simulink model "SimPIDdir2020b"  (R2021b)
settings: Solver=VariableStepAuto  StartTime=0.0  StopTime=15  RelTol=1e-3
values from neighbouring files (symbols this model uses):
  g_r = tf(Mod_r)    [dirPID.m]
  Kd = 1.5    [dirPID.m]
  Ki = 0.005    [dirPID.m]
  Kp = 5    [dirPID.m]
libraries: slpidlib x2, simulink x1
settings Model: Creator=danie  LastModifiedBy=Daniel
settings SolverCC: AlgebraicLoopSolver=TrustRegion
settings DebuggingCC: UnconnectedInputMsg=none  UnconnectedOutputMsg=none  UnconnectedLineMsg=none

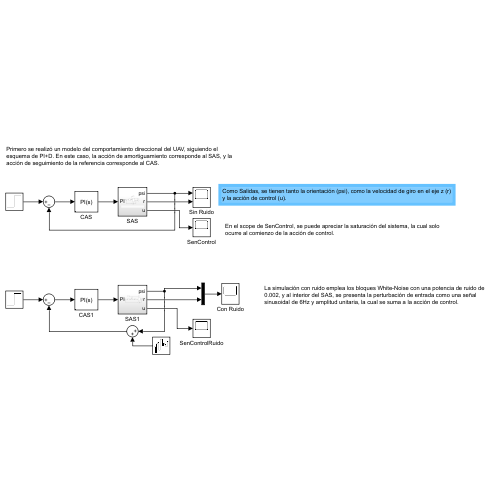
[thumbnail: Simulink's stored preview of the top-level diagram]
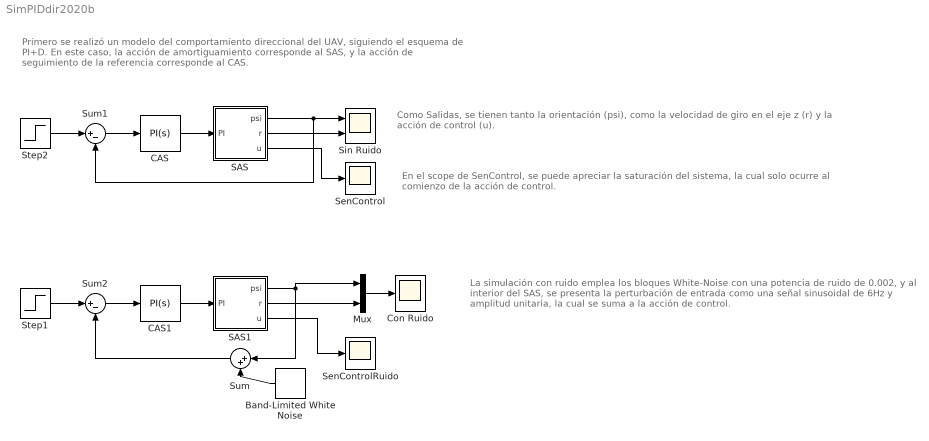
== system SimPIDdir2020b ==
  note: La simulación con ruido emplea los bloques White-Noise con una potencia de ruido de 0.002, y al interior del SAS, se presenta la perturbación de entrada como una señal sinusoidal de 6Hz y amplitud unitaria, la cual se suma a la acción de control.
  note: En el scope de SenControl, se puede apreciar la saturación del sistema, la cual solo ocurre al comienzo de la acción de control.
  note: Como Salidas, se tienen tanto la orientación (psi), como la velocidad de giro en el eje z (r) y la acción de control (u).
  note: Primero se realizó un modelo del comportamiento direccional del UAV, siguiendo el esquema de PI+D. En este caso, la acción de amortiguamiento corresponde al SAS, y la acción de seguimiento de la referencia corresponde al CAS.
  Band-Limited White Noise : simulink/Sources/Band-Limited White Noise  Cov=[0.001]  Ts=0.1  seed=[23341]
  CAS : slpidlib/PID Controller  Controller=PI  Form=Parallel  TimeDomain=Continuous-time  UseExternalTs=off  SampleTime=-1  IntegratorMethod=Forward Euler  FilterMethod=Forward Euler  ControllerParametersSource=internal  P=Kp  I=Ki  D=0  UseFilter=on  N=100  TunerSelectOption=Transfer Function Based (PID Tuner App)  InitialConditionSource=internal  InitialConditionForIntegrator=0  InitialConditionForFilter=0  DifferentiatorICPrevScaledInput=0  ExternalReset=none  TrackingMode=off  Kt=1  LimitOutput=off  SatLimitsSource=internal  UpperSaturationLimit=inf  LowerSaturationLimit=-inf  LinearizeAsGain=on  AntiWindupMode=none  Kb=1  POutMin=[]  POutMax=[]  IOutMin=[]  IOutMax=[]  DOutMin=[]  DOutMax=[]  NOutMin=[]  NOutMax=[]  SumOutMin=[]  SumOutMax=[]  SaturationOutMin=[]  SaturationOutMax=[]  PParamMin=[]  PParamMax=[]  IParamMin=[]  IParamMax=[]  DParamMin=[]  DParamMax=[]  NParamMin=[]  NParamMax=[]  KbParamMin=[]  KbParamMax=[]  KtParamMin=[]  KtParamMax=[]  KbOutMin=[]  KbOutMax=[]  KtOutMin=[]  KtOutMax=[]  IntegratorOutMin=[]  IntegratorOutMax=[]  FilterOutMin=[]  FilterOutMax=[]  SumI1OutMin=[]  SumI1OutMax=[]  SumI2OutMin=[]  SumI2OutMax=[]  SumI3OutMin=[]  SumI3OutMax=[]  SumI4OutMin=[]  SumI4OutMax=[]  SumDOutMin=[]  SumDOutMax=[]  DifferentiatorOutMin=[]  DifferentiatorOutMax=[]  FilterDiffOutCoefMin=[]  FilterDiffOutCoefMax=[]  ReciprocalOutMin=[]  ReciprocalOutMax=[]  SumDenOutMin=[]  SumDenOutMax=[]  SumNumOutMin=[]  SumNumOutMax=[]  DivideOutMin=[]  DivideOutMax=[]  UdiffTsProdOutMin=[]  UdiffTsProdOutMax=[]  NTsProdOutMin=[]  NTsProdOutMax=[]  UintegralTsProdOutMin=[]  UintegralTsProdOutMax=[]  UngainTsProdOutMin=[]  UngainTsProdOutMax=[]  IntegratorContinuousStateAttributes=''  IntegratorStateMustResolveToSignalObject=off  IntegratorRTWStateStorageClass=Auto  FilterContinuousStateAttributes=''  FilterStateMustResolveToSignalObject=off  FilterRTWStateStorageClass=Auto  ParallelPVariant=InternalParameters  IdealPVariant=Disabled  IVariant=InternalParameters  DVariant=Disabled  IntegratorVariant=Continuous  SatVariant=Disabled  AWVariant=Passthrough  PCopyVariant=Disabled  TRVariant=Disabled  FdbkBlocksVariant=Forward  IdealPFdbkVariant=Disabled  SatFdbkVariant=Disabled  DerivativeFilterVariant=Disabled  NVariant=Disabled  NCopyVariant=Disabled_SignalSpec  FilterICVariant=Disabled  IntegratorICVariant=InternalICs  ExternalResetVariant=Disabled  TRSumVariant=Passthrough  SumFdbkVariant=Disabled  SumVariant=Sum_PI  TsampFilterVariant=InternalTs  TsampNgainVariant=Passthrough  TsampIntegralVariant=Passthrough  ExternalSaturationOutDataTypeStr=Inherit: Same as second input
  CAS1 : slpidlib/PID Controller  Controller=PI  Form=Parallel  TimeDomain=Continuous-time  UseExternalTs=off  SampleTime=-1  IntegratorMethod=Forward Euler  FilterMethod=Forward Euler  ControllerParametersSource=internal  P=Kp  I=Ki  D=0  UseFilter=on  N=100  TunerSelectOption=Transfer Function Based (PID Tuner App)  InitialConditionSource=internal  InitialConditionForIntegrator=0  InitialConditionForFilter=0  DifferentiatorICPrevScaledInput=0  ExternalReset=none  TrackingMode=off  Kt=1  LimitOutput=off  SatLimitsSource=internal  UpperSaturationLimit=inf  LowerSaturationLimit=-inf  LinearizeAsGain=on  AntiWindupMode=none  Kb=1  POutMin=[]  POutMax=[]  IOutMin=[]  IOutMax=[]  DOutMin=[]  DOutMax=[]  NOutMin=[]  NOutMax=[]  SumOutMin=[]  SumOutMax=[]  SaturationOutMin=[]  SaturationOutMax=[]  PParamMin=[]  PParamMax=[]  IParamMin=[]  IParamMax=[]  DParamMin=[]  DParamMax=[]  NParamMin=[]  NParamMax=[]  KbParamMin=[]  KbParamMax=[]  KtParamMin=[]  KtParamMax=[]  KbOutMin=[]  KbOutMax=[]  KtOutMin=[]  KtOutMax=[]  IntegratorOutMin=[]  IntegratorOutMax=[]  FilterOutMin=[]  FilterOutMax=[]  SumI1OutMin=[]  SumI1OutMax=[]  SumI2OutMin=[]  SumI2OutMax=[]  SumI3OutMin=[]  SumI3OutMax=[]  SumI4OutMin=[]  SumI4OutMax=[]  SumDOutMin=[]  SumDOutMax=[]  DifferentiatorOutMin=[]  DifferentiatorOutMax=[]  FilterDiffOutCoefMin=[]  FilterDiffOutCoefMax=[]  ReciprocalOutMin=[]  ReciprocalOutMax=[]  SumDenOutMin=[]  SumDenOutMax=[]  SumNumOutMin=[]  SumNumOutMax=[]  DivideOutMin=[]  DivideOutMax=[]  UdiffTsProdOutMin=[]  UdiffTsProdOutMax=[]  NTsProdOutMin=[]  NTsProdOutMax=[]  UintegralTsProdOutMin=[]  UintegralTsProdOutMax=[]  UngainTsProdOutMin=[]  UngainTsProdOutMax=[]  IntegratorContinuousStateAttributes=''  IntegratorStateMustResolveToSignalObject=off  IntegratorRTWStateStorageClass=Auto  FilterContinuousStateAttributes=''  FilterStateMustResolveToSignalObject=off  FilterRTWStateStorageClass=Auto  ParallelPVariant=InternalParameters  IdealPVariant=Disabled  IVariant=InternalParameters  DVariant=Disabled  IntegratorVariant=Continuous  SatVariant=Disabled  AWVariant=Passthrough  PCopyVariant=Disabled  TRVariant=Disabled  FdbkBlocksVariant=Forward  IdealPFdbkVariant=Disabled  SatFdbkVariant=Disabled  DerivativeFilterVariant=Disabled  NVariant=Disabled  NCopyVariant=Disabled_SignalSpec  FilterICVariant=Disabled  IntegratorICVariant=InternalICs  ExternalResetVariant=Disabled  TRSumVariant=Passthrough  SumFdbkVariant=Disabled  SumVariant=Sum_PI  TsampFilterVariant=InternalTs  TsampNgainVariant=Passthrough  TsampIntegralVariant=Passthrough  ExternalSaturationOutDataTypeStr=Inherit: Same as second input
  Con Ruido : Scope
  Mux : Mux  Inputs=2
  SAS : Subsystem
  SAS1 : Subsystem
  SenControl : Scope
  SenControlRuido : Scope
  Sin Ruido : Scope  NumInputPorts=2
  Step1 : Step  Time=0  After=40  SampleTime=0
  Step2 : Step  Time=0  After=40  SampleTime=0
  Sum : Sum  Inputs=|++
  Sum1 : Sum  Inputs=|+-
  Sum2 : Sum  Inputs=|+-
  wires:
  Sum1/1 -> CAS/1
  SAS/1(psi) -> Sin Ruido/1, Sum1/2
  CAS/1 -> SAS/1(PI)
  Step2/1 -> Sum1/1
  Step1/1 -> Sum2/1
  CAS1/1 -> SAS1/1(PI)
  SAS1/2(r) -> Mux/2
  SAS1/1(psi) -> Mux/1, Sum/1
  Sum2/1 -> CAS1/1
  Band-Limited White Noise/1 -> Sum/2
  Sum/1 -> Sum2/2
  SAS/3(u) -> SenControl/1
  SAS1/3(u) -> SenControlRuido/1
  SAS/2(r) -> Sin Ruido/2
  Mux/1 -> Con Ruido/1

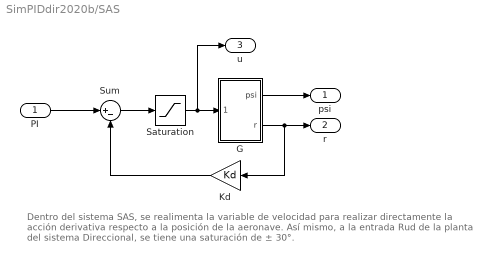
== system SimPIDdir2020b/SAS ==
  note: Dentro del sistema SAS, se realimenta la variable de velocidad para realizar directamente la acción derivativa respecto a la posición de la aeronave. Así mismo, a la entrada Rud de la planta del sistema Direccional, se tiene una saturación de ± 30°.
  PI : Inport
  G : Subsystem
  Kd : Gain  Gain=Kd
  Saturation : Saturate  UpperLimit=30  LowerLimit=-30
  Sum : Sum  Inputs=|+-
  psi : Outport
  r : Outport  Port=2
  u : Outport  Port=3
  wires:
  G/2(r) -> r/1, Kd/1
  Kd/1 -> Sum/2
  G/1(psi) -> psi/1
  Sum/1 -> Saturation/1
  PI/1 -> Sum/1
  Saturation/1 -> u/1, G/1(Rud)

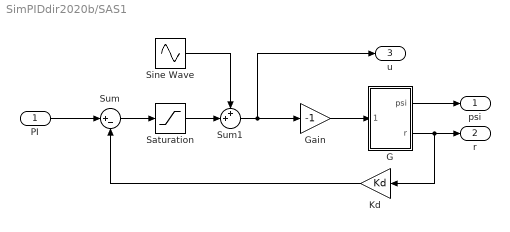
== system SimPIDdir2020b/SAS1 ==
  PI : Inport
  G : Subsystem
  Gain : Gain  Gain=-1
  Kd : Gain  Gain=Kd
  Saturation : Saturate  UpperLimit=30  LowerLimit=-30
  Sine Wave : Sin  Frequency=12*pi  SampleTime=0
  Sum : Sum  Inputs=|+-
  Sum1 : Sum  Inputs=++|
  psi : Outport
  r : Outport  Port=2
  u : Outport  Port=3
  wires:
  PI/1 -> Sum/1
  Sum/1 -> Saturation/1
  G/1(psi) -> psi/1
  Kd/1 -> Sum/2
  G/2(r) -> Kd/1, r/1
  Saturation/1 -> Sum1/2
  Sum1/1 -> u/1, Gain/1
  Sine Wave/1 -> Sum1/1
  Gain/1 -> G/1(Rud)

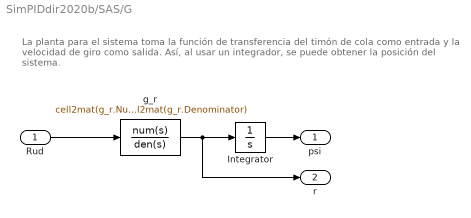
== system SimPIDdir2020b/SAS/G ==
  note: La planta para el sistema toma la función de transferencia del timón de cola como entrada y la velocidad de giro como salida. Así, al usar un integrador, se puede obtener la posición del sistema.
  Rud : Inport
  Integrator : Integrator
  g_r : TransferFcn  Numerator=cell2mat(g_r.Numerator)  Denominator=cell2mat(g_r.Denominator)
  psi : Outport
  r : Outport  Port=2
  wires:
  g_r/1 -> r/1, Integrator/1
  Integrator/1 -> psi/1
  Rud/1 -> g_r/1

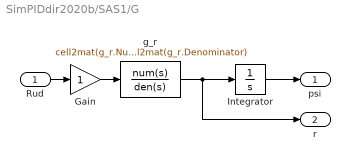
== system SimPIDdir2020b/SAS1/G ==
  Rud : Inport
  Gain : Gain
  Integrator : Integrator
  g_r : TransferFcn  Numerator=cell2mat(g_r.Numerator)  Denominator=cell2mat(g_r.Denominator)
  psi : Outport
  r : Outport  Port=2
  wires:
  Rud/1 -> Gain/1
  Gain/1 -> g_r/1
  Integrator/1 -> psi/1
  g_r/1 -> Integrator/1, r/1
